simulink model "ADC_Model_Single_Phase"  (R2018a)
settings: configuration reference "ModelConfig_var" (kept outside this file)
model workspace (MAT data in the model file):
  ADCBit_I = 1
  ADCBit_V = 1
  Gain_I = 1
  Gain_V = 1
  Offset_I = 1
  Offset_V = 1
  Out_mode_I = 1
  Out_mode_V = 1
  PGA_Gain_I = 1
  PGA_Gain_V = 1
  Vcc_I = 1
  Vcc_V = 1
settings Model: ParameterArgumentNames=ADCBit_I,ADCBit_V,Gain_I,Gain_V,Offset_I,Offset_V,Out_mode_I,Out_mode_V,PGA_Gain_I,PGA_Gain_V,Vcc_I,Vcc_V  OrderedModelArguments=off  Creator=BEDNASA  LastModifiedBy=BEDNASA
settings ConfigSetRef: SourceLocation=Base Workspace

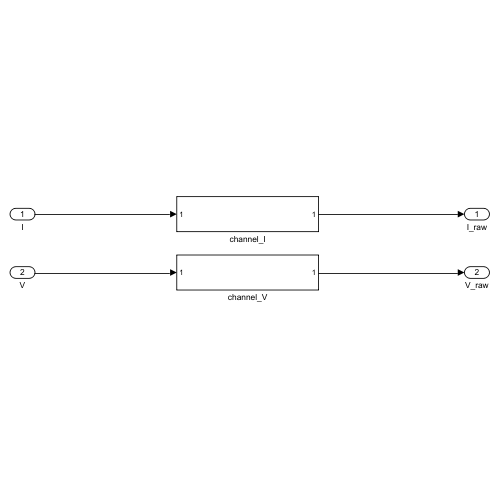
[thumbnail: Simulink's stored preview of the top-level diagram]
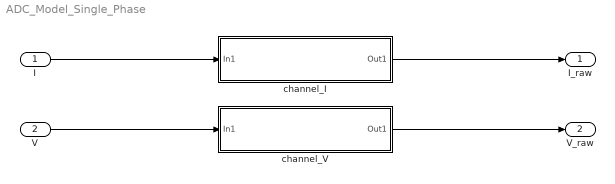
== system ADC_Model_Single_Phase ==
  I : Inport
  V : Inport  Port=2
  channel_I : Subsystem  mask(ADC model){Out_Mode=Out_mode_I, Gain=Gain_I, Offset=Offset_I, Vcc=Vcc_I, ADCBit=ADCBit_I, PGA_Gain=PGA_Gain_I}
      mask prompts: Out_Mode "Output Mode"
      mask help: Atomic ADC model utlized in custom blocks for single and three phase drive systems
      mask TypeOptions Out_Mode: MATLAB Function/Out_Mode
      mask TypeOptions Gain: MATLAB Function/Gain
      mask TypeOptions Offset: MATLAB Function/Offset
      mask TypeOptions Vcc: MATLAB Function/Vcc
      mask TypeOptions ADCBit: MATLAB Function/ADCBit
      mask TypeOptions PGA_Gain: MATLAB Function/PGA_Gain
      mask DialogControl Container3 Prompt: SIL (0) \ RT PIL (1)
  channel_V : Subsystem  mask(ADC model){Out_Mode=Out_mode_V, Gain=Gain_V, Offset=Offset_V, Vcc=Vcc_V, ADCBit=ADCBit_V, PGA_Gain=PGA_Gain_V}
      mask prompts: Out_Mode "Output Mode"
      mask help: Atomic ADC model utlized in custom blocks for single and three phase drive systems
      mask TypeOptions Out_Mode: MATLAB Function/Out_Mode
      mask TypeOptions Gain: MATLAB Function/Gain
      mask TypeOptions Offset: MATLAB Function/Offset
      mask TypeOptions Vcc: MATLAB Function/Vcc
      mask TypeOptions ADCBit: MATLAB Function/ADCBit
      mask TypeOptions PGA_Gain: MATLAB Function/PGA_Gain
      mask DialogControl Container3 Prompt: SIL (0) \ RT PIL (1)
  I_raw : Outport
  V_raw : Outport  Port=2
  wires:
  V/1 -> channel_V/1(In1)
  channel_V/1(Out1) -> V_raw/1
  channel_I/1(Out1) -> I_raw/1
  I/1 -> channel_I/1(In1)

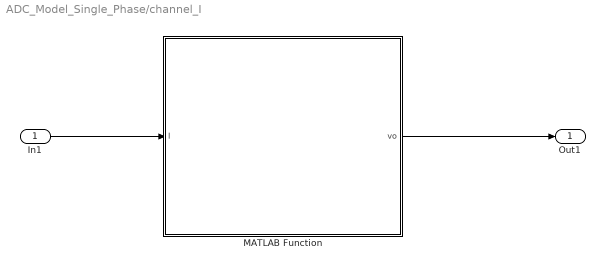
== system ADC_Model_Single_Phase/channel_I ==
  In1 : Inport
  MATLAB Function : MATLAB Function  TreatAsAtomicUnit=on  mask(ADC model){Out_Mode=Out_Mode, Gain=Gain, Offset=Offset, Vcc=Vcc, ADCBit=ADCBit, PGA_Gain=PGA_Gain}
      mask prompts: Out_Mode "Output Mode"
      mask help: Atomic ADC model utlized in custom blocks for single and three phase drive systems
  Out1 : Outport
  wires:
  In1/1 -> MATLAB Function/1(I)
  MATLAB Function/1(vo) -> Out1/1

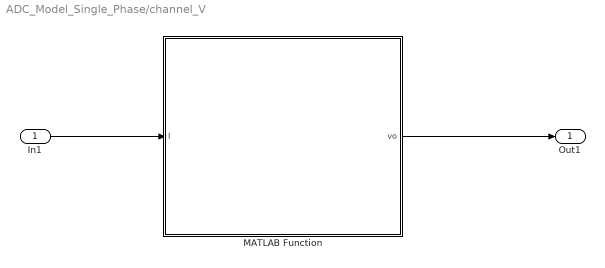
== system ADC_Model_Single_Phase/channel_V ==
  In1 : Inport
  MATLAB Function : MATLAB Function  TreatAsAtomicUnit=on  mask(ADC model){Out_Mode=Out_Mode, Gain=Gain, Offset=Offset, Vcc=Vcc, ADCBit=ADCBit, PGA_Gain=PGA_Gain}
      mask prompts: Out_Mode "Output Mode"
      mask help: Atomic ADC model utlized in custom blocks for single and three phase drive systems
  Out1 : Outport
  wires:
  In1/1 -> MATLAB Function/1(I)
  MATLAB Function/1(vo) -> Out1/1

== matlab function ADC_Model_Single_Phase/channel_V/MATLAB Function ==
  data: I input; vo output; Gain parameter; Offset parameter; Vcc parameter; ADCBit parameter; PGA_Gain parameter; Out_Mode parameter
function vo = GetADCRawData(I, Gain, Offset, Vcc, ADCBit, PGA_Gain, Out_Mode)

%Vcc = 1;
%out_mode = 0;
%ADCBit = 12;


%Vout = C1*I+C2;
%Vout_PIL = 1;

Vout=Gain * I + Offset;
Vout_PIL = (Gain/PGA_Gain) * I + Offset/PGA_Gain;

if (Vout > Vcc)
    Vout = Vcc;
elseif (Vout < 0)
    Vout = 0;
end

if Out_Mode == 0        % ADC_counts
    vo = round((Vout/Vcc) * (2^ADCBit));
elseif Out_Mode == 1    % ADC_voltage
    vo = Vout_PIL;
else 
    vo = 0;
end


% function AD_count  = GetADCRawData(in_analog, Gain, Offset, Vcc, ADCbit)
% %% Sensor model with ADC
% % Sensor voltage equation V_out = Gain * in_analog + Offset
% 
% V_out = Gain * in_analog + Offset;
% 
% if (V_out > Vcc)
%     V_out = Vcc;
% elseif (V_out < 0)
%     V_out = 0;
% end
% 
% %% AD Counts
% AD_count = round((V_out/Vcc) * (2^ADCbit));
% end

== matlab function ADC_Model_Single_Phase/channel_I/MATLAB Function ==
  data: I input; vo output; Gain parameter; Offset parameter; Vcc parameter; ADCBit parameter; PGA_Gain parameter; Out_Mode parameter
function vo = GetADCRawData(I, Gain, Offset, Vcc, ADCBit, PGA_Gain, Out_Mode)

%Vcc = 1;
%out_mode = 0;
%ADCBit = 12;


%Vout = C1*I+C2;
%Vout_PIL = 1;

Vout=Gain * I + Offset;
Vout_PIL = (Gain/PGA_Gain) * I + Offset/PGA_Gain;

if (Vout > Vcc)
    Vout = Vcc;
elseif (Vout < 0)
    Vout = 0;
end

if Out_Mode == 0        % ADC_counts
    vo = round((Vout/Vcc) * (2^ADCBit));
elseif Out_Mode == 1    % ADC_voltage
    vo = Vout_PIL;
else 
    vo = 0;
end


% function AD_count  = GetADCRawData(in_analog, Gain, Offset, Vcc, ADCbit)
% %% Sensor model with ADC
% % Sensor voltage equation V_out = Gain * in_analog + Offset
% 
% V_out = Gain * in_analog + Offset;
% 
% if (V_out > Vcc)
%     V_out = Vcc;
% elseif (V_out < 0)
%     V_out = 0;
% end
% 
% %% AD Counts
% AD_count = round((V_out/Vcc) * (2^ADCbit));
% end
